simulink model "xblock_half_band_Model"  (Simulink 7.4)
settings: Solver=ode45  StartTime=0.0  StopTime=10.0  RelTol=1e-3
libraries: xbsIndex_r4 x629, casper_library_misc x12
(part 2 of 6)

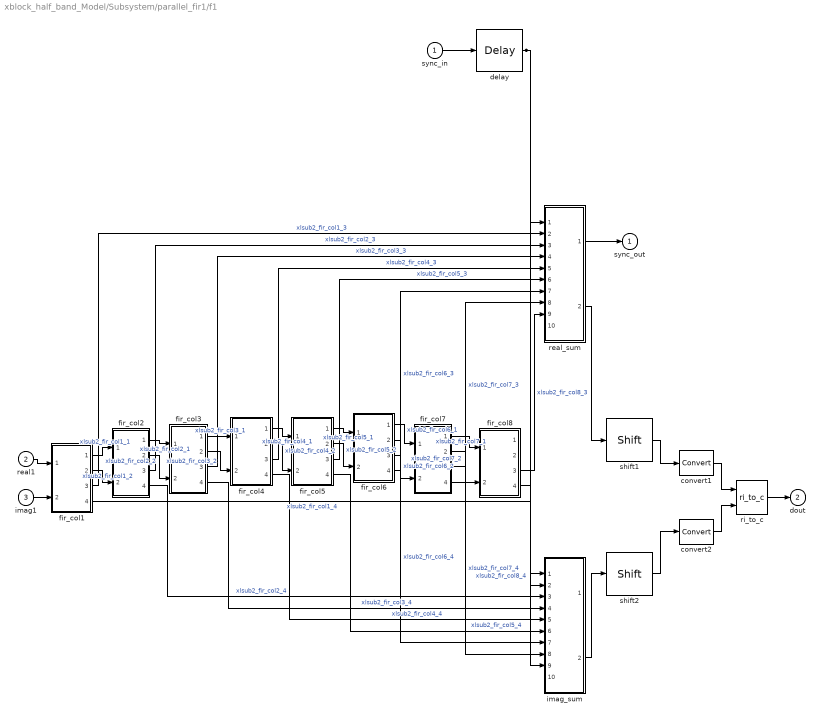
== system xblock_half_band_Model/Subsystem/parallel_fir1/f1 ==
  sync_in : Inport
  real1 : Inport  Port=2
  imag1 : Inport  Port=3
  convert1 : xbsIndex_r4/Convert  arith_type="Signed  (2's comp)"  n_bits=4  bin_pt=3  quantization=Truncate  overflow=Wrap  latency=1  dbl_ovrd=off  pipeline=off  block_type=convert
      settings: block_version=11.4
  convert2 : xbsIndex_r4/Convert  arith_type="Signed  (2's comp)"  n_bits=4  bin_pt=3  quantization=Truncate  overflow=Wrap  latency=1  dbl_ovrd=off  pipeline=off  block_type=convert
      settings: block_version=11.4
  delay : xbsIndex_r4/Delay  en=off  latency=3  dbl_ovrd=off  reg_retiming=off  block_type=delay
      settings: block_version=11.4
  fir_col1 : Subsystem
  fir_col2 : Subsystem
  fir_col3 : Subsystem
  fir_col4 : Subsystem
  fir_col5 : Subsystem
  fir_col6 : Subsystem
  fir_col7 : Subsystem
  fir_col8 : Subsystem
  imag_sum : Subsystem
  real_sum : Subsystem
  ri_to_c : casper_library_misc/ri_to_c  SystemSampleTime=-1
  shift1 : xbsIndex_r4/Shift  shift_dir=Left  shift_bits=1  en=off  latency=0  precision=Full  arith_type="Signed  (2's comp)"  n_bits=16  bin_pt=14  quantization=Truncate  overflow=Wrap  dbl_ovrd=off  block_type=shift
  shift2 : xbsIndex_r4/Shift  shift_dir=Left  shift_bits=1  en=off  latency=0  precision=Full  arith_type="Signed  (2's comp)"  n_bits=16  bin_pt=14  quantization=Truncate  overflow=Wrap  dbl_ovrd=off  block_type=shift
  sync_out : Outport
  dout : Outport  Port=2
  wires:
  delay/1 -> real_sum/1(sync), imag_sum/1(sync)
  imag_sum/2(dout) -> shift2/1
  shift1/1 -> convert1/1
  convert2/1 -> ri_to_c/2
  fir_col8/3(real_sum) -> real_sum/9(din_8)  "xlsub2_fir_col8_3"
  fir_col6/3(real_sum) -> real_sum/7(din_6)  "xlsub2_fir_col6_3"
  fir_col4/3(real_sum) -> real_sum/5(din_4)  "xlsub2_fir_col4_3"
  fir_col2/3(real_sum) -> real_sum/3(din_2)  "xlsub2_fir_col2_3"
  fir_col8/4(imag_sum) -> imag_sum/9(din_8)  "xlsub2_fir_col8_4"
  fir_col6/4(imag_sum) -> imag_sum/7(din_6)  "xlsub2_fir_col6_4"
  fir_col4/4(imag_sum) -> imag_sum/5(din_4)  "xlsub2_fir_col4_4"
  fir_col2/4(imag_sum) -> imag_sum/3(din_2)  "xlsub2_fir_col2_4"
  fir_col7/2(imag_out1) -> fir_col8/2(imag1)  "xlsub2_fir_col7_2"
  fir_col6/1(real_out1) -> fir_col7/1(real1)  "xlsub2_fir_col6_1"
  fir_col5/2(imag_out1) -> fir_col6/2(imag1)  "xlsub2_fir_col5_2"
  fir_col4/1(real_out1) -> fir_col5/1(real1)  "xlsub2_fir_col4_1"
  fir_col3/2(imag_out1) -> fir_col4/2(imag1)  "xlsub2_fir_col3_2"
  fir_col2/1(real_out1) -> fir_col3/1(real1)  "xlsub2_fir_col2_1"
  fir_col1/2(imag_out1) -> fir_col2/2(imag1)  "xlsub2_fir_col1_2"
  real1/1 -> fir_col1/1(real1)
  sync_in/1 -> delay/1
  imag1/1 -> fir_col1/2(imag1)
  fir_col1/1(real_out1) -> fir_col2/1(real1)  "xlsub2_fir_col1_1"
  fir_col2/2(imag_out1) -> fir_col3/2(imag1)  "xlsub2_fir_col2_2"
  fir_col3/1(real_out1) -> fir_col4/1(real1)  "xlsub2_fir_col3_1"
  fir_col4/2(imag_out1) -> fir_col5/2(imag1)  "xlsub2_fir_col4_2"
  fir_col5/1(real_out1) -> fir_col6/1(real1)  "xlsub2_fir_col5_1"
  fir_col6/2(imag_out1) -> fir_col7/2(imag1)  "xlsub2_fir_col6_2"
  fir_col7/1(real_out1) -> fir_col8/1(real1)  "xlsub2_fir_col7_1"
  fir_col1/4(imag_sum) -> imag_sum/2(din_1)  "xlsub2_fir_col1_4"
  fir_col3/4(imag_sum) -> imag_sum/4(din_3)  "xlsub2_fir_col3_4"
  fir_col5/4(imag_sum) -> imag_sum/6(din_5)  "xlsub2_fir_col5_4"
  fir_col7/4(imag_sum) -> imag_sum/8(din_7)  "xlsub2_fir_col7_4"
  fir_col1/3(real_sum) -> real_sum/2(din_1)  "xlsub2_fir_col1_3"
  fir_col3/3(real_sum) -> real_sum/4(din_3)  "xlsub2_fir_col3_3"
  fir_col5/3(real_sum) -> real_sum/6(din_5)  "xlsub2_fir_col5_3"
  fir_col7/3(real_sum) -> real_sum/8(din_7)  "xlsub2_fir_col7_3"
  real_sum/1(sync_out) -> sync_out/1
  convert1/1 -> ri_to_c/1
  ri_to_c/1 -> dout/1
  real_sum/2(dout) -> shift1/1
  shift2/1 -> convert2/1

== system xblock_half_band_Model/Subsystem/parallel_fir2/c_to_ri ==
  c : Inport
  force_im : xbsIndex_r4/Reinterpret  force_arith_type=on  arith_type="Signed  (2's comp)"  force_bin_pt=on  bin_pt=7  block_type=reinterpret
      settings: infoedit="Changes signal type without altering the binary representation.   You can changed the signal between signed and unsigned, and relocate the binary point.<br><br>Hardware notes: In hardware this block costs nothing.<br><br>Example:  Suppose the input is 6 bits wide, signed, with 2 fractional bits, and the output is forced to unsigned with 0 fractional bits.  Then an input of -2.0 (1110.00 in binary 2's complement) becomes an output of 56 (111000 in binary)."
  force_re : xbsIndex_r4/Reinterpret  force_arith_type=on  arith_type="Signed  (2's comp)"  force_bin_pt=on  bin_pt=7  block_type=reinterpret
      settings: infoedit="Changes signal type without altering the binary representation.   You can changed the signal between signed and unsigned, and relocate the binary point.<br><br>Hardware notes: In hardware this block costs nothing.<br><br>Example:  Suppose the input is 6 bits wide, signed, with 2 fractional bits, and the output is forced to unsigned with 0 fractional bits.  Then an input of -2.0 (1110.00 in binary 2's complement) becomes an output of 56 (111000 in binary)."
  slice_im : xbsIndex_r4/Slice  nbits=8  boolean_output=off  mode=Lower Bit Location + Width  bit1=0  base1=MSB of Input  bit0=0  base0=LSB of Input  dbl_ovrd=off  block_type=slice
  slice_re : xbsIndex_r4/Slice  nbits=8  boolean_output=off  mode=Upper Bit Location + Width  bit1=0  base1=MSB of Input  bit0=0  base0=LSB of Input  dbl_ovrd=off  block_type=slice
  re : Outport
  im : Outport  Port=2
  wires:
  c/1 -> slice_re/1, slice_im/1
  slice_im/1 -> force_im/1
  force_im/1 -> im/1
  force_re/1 -> re/1
  slice_re/1 -> force_re/1

== system xblock_half_band_Model/Subsystem/parallel_fir2/c_to_ri1 ==
  c : Inport
  force_im : xbsIndex_r4/Reinterpret  force_arith_type=on  arith_type="Signed  (2's comp)"  force_bin_pt=on  bin_pt=7  block_type=reinterpret
      settings: infoedit="Changes signal type without altering the binary representation.   You can changed the signal between signed and unsigned, and relocate the binary point.<br><br>Hardware notes: In hardware this block costs nothing.<br><br>Example:  Suppose the input is 6 bits wide, signed, with 2 fractional bits, and the output is forced to unsigned with 0 fractional bits.  Then an input of -2.0 (1110.00 in binary 2's complement) becomes an output of 56 (111000 in binary)."
  force_re : xbsIndex_r4/Reinterpret  force_arith_type=on  arith_type="Signed  (2's comp)"  force_bin_pt=on  bin_pt=7  block_type=reinterpret
      settings: infoedit="Changes signal type without altering the binary representation.   You can changed the signal between signed and unsigned, and relocate the binary point.<br><br>Hardware notes: In hardware this block costs nothing.<br><br>Example:  Suppose the input is 6 bits wide, signed, with 2 fractional bits, and the output is forced to unsigned with 0 fractional bits.  Then an input of -2.0 (1110.00 in binary 2's complement) becomes an output of 56 (111000 in binary)."
  slice_im : xbsIndex_r4/Slice  nbits=8  boolean_output=off  mode=Lower Bit Location + Width  bit1=0  base1=MSB of Input  bit0=0  base0=LSB of Input  dbl_ovrd=off  block_type=slice
  slice_re : xbsIndex_r4/Slice  nbits=8  boolean_output=off  mode=Upper Bit Location + Width  bit1=0  base1=MSB of Input  bit0=0  base0=LSB of Input  dbl_ovrd=off  block_type=slice
  re : Outport
  im : Outport  Port=2
  wires:
  c/1 -> slice_re/1, slice_im/1
  slice_im/1 -> force_im/1
  force_im/1 -> im/1
  force_re/1 -> re/1
  slice_re/1 -> force_re/1

== system xblock_half_band_Model/Subsystem/parallel_fir2/c_to_ri2 ==
  c : Inport
  force_im : xbsIndex_r4/Reinterpret  force_arith_type=on  arith_type="Signed  (2's comp)"  force_bin_pt=on  bin_pt=7  block_type=reinterpret
      settings: infoedit="Changes signal type without altering the binary representation.   You can changed the signal between signed and unsigned, and relocate the binary point.<br><br>Hardware notes: In hardware this block costs nothing.<br><br>Example:  Suppose the input is 6 bits wide, signed, with 2 fractional bits, and the output is forced to unsigned with 0 fractional bits.  Then an input of -2.0 (1110.00 in binary 2's complement) becomes an output of 56 (111000 in binary)."
  force_re : xbsIndex_r4/Reinterpret  force_arith_type=on  arith_type="Signed  (2's comp)"  force_bin_pt=on  bin_pt=7  block_type=reinterpret
      settings: infoedit="Changes signal type without altering the binary representation.   You can changed the signal between signed and unsigned, and relocate the binary point.<br><br>Hardware notes: In hardware this block costs nothing.<br><br>Example:  Suppose the input is 6 bits wide, signed, with 2 fractional bits, and the output is forced to unsigned with 0 fractional bits.  Then an input of -2.0 (1110.00 in binary 2's complement) becomes an output of 56 (111000 in binary)."
  slice_im : xbsIndex_r4/Slice  nbits=8  boolean_output=off  mode=Lower Bit Location + Width  bit1=0  base1=MSB of Input  bit0=0  base0=LSB of Input  dbl_ovrd=off  block_type=slice
  slice_re : xbsIndex_r4/Slice  nbits=8  boolean_output=off  mode=Upper Bit Location + Width  bit1=0  base1=MSB of Input  bit0=0  base0=LSB of Input  dbl_ovrd=off  block_type=slice
  re : Outport
  im : Outport  Port=2
  wires:
  c/1 -> slice_re/1, slice_im/1
  slice_im/1 -> force_im/1
  force_im/1 -> im/1
  force_re/1 -> re/1
  slice_re/1 -> force_re/1

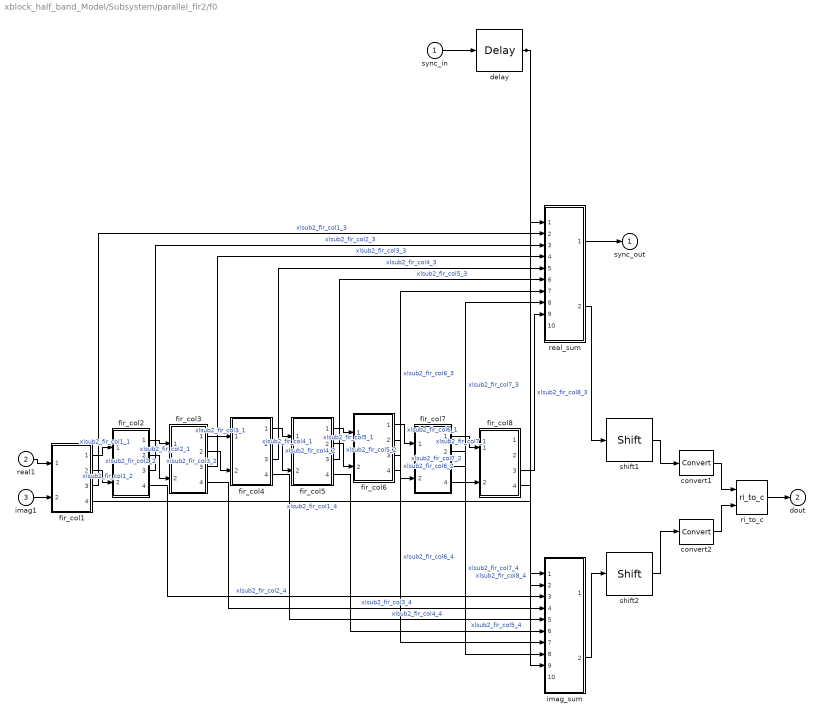
== system xblock_half_band_Model/Subsystem/parallel_fir2/f0 ==
  sync_in : Inport
  real1 : Inport  Port=2
  imag1 : Inport  Port=3
  convert1 : xbsIndex_r4/Convert  arith_type="Signed  (2's comp)"  n_bits=4  bin_pt=3  quantization=Truncate  overflow=Wrap  latency=1  dbl_ovrd=off  pipeline=off  block_type=convert
      settings: block_version=11.4
  convert2 : xbsIndex_r4/Convert  arith_type="Signed  (2's comp)"  n_bits=4  bin_pt=3  quantization=Truncate  overflow=Wrap  latency=1  dbl_ovrd=off  pipeline=off  block_type=convert
      settings: block_version=11.4
  delay : xbsIndex_r4/Delay  en=off  latency=3  dbl_ovrd=off  reg_retiming=off  block_type=delay
      settings: block_version=11.4
  fir_col1 : Subsystem
  fir_col2 : Subsystem
  fir_col3 : Subsystem
  fir_col4 : Subsystem
  fir_col5 : Subsystem
  fir_col6 : Subsystem
  fir_col7 : Subsystem
  fir_col8 : Subsystem
  imag_sum : Subsystem
  real_sum : Subsystem
  ri_to_c : casper_library_misc/ri_to_c  SystemSampleTime=-1
  shift1 : xbsIndex_r4/Shift  shift_dir=Left  shift_bits=1  en=off  latency=0  precision=Full  arith_type="Signed  (2's comp)"  n_bits=16  bin_pt=14  quantization=Truncate  overflow=Wrap  dbl_ovrd=off  block_type=shift
  shift2 : xbsIndex_r4/Shift  shift_dir=Left  shift_bits=1  en=off  latency=0  precision=Full  arith_type="Signed  (2's comp)"  n_bits=16  bin_pt=14  quantization=Truncate  overflow=Wrap  dbl_ovrd=off  block_type=shift
  sync_out : Outport
  dout : Outport  Port=2
  wires:
  delay/1 -> real_sum/1(sync), imag_sum/1(sync)
  imag_sum/2(dout) -> shift2/1
  shift1/1 -> convert1/1
  convert2/1 -> ri_to_c/2
  fir_col8/3(real_sum) -> real_sum/9(din_8)  "xlsub2_fir_col8_3"
  fir_col6/3(real_sum) -> real_sum/7(din_6)  "xlsub2_fir_col6_3"
  fir_col4/3(real_sum) -> real_sum/5(din_4)  "xlsub2_fir_col4_3"
  fir_col2/3(real_sum) -> real_sum/3(din_2)  "xlsub2_fir_col2_3"
  fir_col8/4(imag_sum) -> imag_sum/9(din_8)  "xlsub2_fir_col8_4"
  fir_col6/4(imag_sum) -> imag_sum/7(din_6)  "xlsub2_fir_col6_4"
  fir_col4/4(imag_sum) -> imag_sum/5(din_4)  "xlsub2_fir_col4_4"
  fir_col2/4(imag_sum) -> imag_sum/3(din_2)  "xlsub2_fir_col2_4"
  fir_col7/2(imag_out1) -> fir_col8/2(imag1)  "xlsub2_fir_col7_2"
  fir_col6/1(real_out1) -> fir_col7/1(real1)  "xlsub2_fir_col6_1"
  fir_col5/2(imag_out1) -> fir_col6/2(imag1)  "xlsub2_fir_col5_2"
  fir_col4/1(real_out1) -> fir_col5/1(real1)  "xlsub2_fir_col4_1"
  fir_col3/2(imag_out1) -> fir_col4/2(imag1)  "xlsub2_fir_col3_2"
  fir_col2/1(real_out1) -> fir_col3/1(real1)  "xlsub2_fir_col2_1"
  fir_col1/2(imag_out1) -> fir_col2/2(imag1)  "xlsub2_fir_col1_2"
  real1/1 -> fir_col1/1(real1)
  sync_in/1 -> delay/1
  imag1/1 -> fir_col1/2(imag1)
  fir_col1/1(real_out1) -> fir_col2/1(real1)  "xlsub2_fir_col1_1"
  fir_col2/2(imag_out1) -> fir_col3/2(imag1)  "xlsub2_fir_col2_2"
  fir_col3/1(real_out1) -> fir_col4/1(real1)  "xlsub2_fir_col3_1"
  fir_col4/2(imag_out1) -> fir_col5/2(imag1)  "xlsub2_fir_col4_2"
  fir_col5/1(real_out1) -> fir_col6/1(real1)  "xlsub2_fir_col5_1"
  fir_col6/2(imag_out1) -> fir_col7/2(imag1)  "xlsub2_fir_col6_2"
  fir_col7/1(real_out1) -> fir_col8/1(real1)  "xlsub2_fir_col7_1"
  fir_col1/4(imag_sum) -> imag_sum/2(din_1)  "xlsub2_fir_col1_4"
  fir_col3/4(imag_sum) -> imag_sum/4(din_3)  "xlsub2_fir_col3_4"
  fir_col5/4(imag_sum) -> imag_sum/6(din_5)  "xlsub2_fir_col5_4"
  fir_col7/4(imag_sum) -> imag_sum/8(din_7)  "xlsub2_fir_col7_4"
  fir_col1/3(real_sum) -> real_sum/2(din_1)  "xlsub2_fir_col1_3"
  fir_col3/3(real_sum) -> real_sum/4(din_3)  "xlsub2_fir_col3_3"
  fir_col5/3(real_sum) -> real_sum/6(din_5)  "xlsub2_fir_col5_3"
  fir_col7/3(real_sum) -> real_sum/8(din_7)  "xlsub2_fir_col7_3"
  real_sum/1(sync_out) -> sync_out/1
  convert1/1 -> ri_to_c/1
  ri_to_c/1 -> dout/1
  real_sum/2(dout) -> shift1/1
  shift2/1 -> convert2/1

== system xblock_half_band_Model/Subsystem/parallel_fir2/f0pf1 ==
  sync_in : Inport
  real1 : Inport  Port=2
  imag1 : Inport  Port=3
  convert1 : xbsIndex_r4/Convert  arith_type="Signed  (2's comp)"  n_bits=4  bin_pt=3  quantization=Truncate  overflow=Wrap  latency=1  dbl_ovrd=off  pipeline=off  block_type=convert
      settings: block_version=11.4
  convert2 : xbsIndex_r4/Convert  arith_type="Signed  (2's comp)"  n_bits=4  bin_pt=3  quantization=Truncate  overflow=Wrap  latency=1  dbl_ovrd=off  pipeline=off  block_type=convert
      settings: block_version=11.4
  delay : xbsIndex_r4/Delay  en=off  latency=3  dbl_ovrd=off  reg_retiming=off  block_type=delay
      settings: block_version=11.4
  fir_col1 : Subsystem
  fir_col2 : Subsystem
  fir_col3 : Subsystem
  fir_col4 : Subsystem
  fir_col5 : Subsystem
  imag_sum : Subsystem
  real_sum : Subsystem
  ri_to_c : casper_library_misc/ri_to_c  SystemSampleTime=-1
  shift1 : xbsIndex_r4/Shift  shift_dir=Left  shift_bits=1  en=off  latency=0  precision=Full  arith_type="Signed  (2's comp)"  n_bits=16  bin_pt=14  quantization=Truncate  overflow=Wrap  dbl_ovrd=off  block_type=shift
  shift2 : xbsIndex_r4/Shift  shift_dir=Left  shift_bits=1  en=off  latency=0  precision=Full  arith_type="Signed  (2's comp)"  n_bits=16  bin_pt=14  quantization=Truncate  overflow=Wrap  dbl_ovrd=off  block_type=shift
  sync_out : Outport
  dout : Outport  Port=2
  wires:
  delay/1 -> imag_sum/1(sync), real_sum/1(sync)
  imag_sum/2(dout) -> shift2/1
  shift1/1 -> convert1/1
  convert2/1 -> ri_to_c/2
  fir_col5/3(real_sum) -> real_sum/6(din_5)  "xlsub2_fir_col5_3"
  fir_col3/3(real_sum) -> real_sum/4(din_3)  "xlsub2_fir_col3_3"
  fir_col1/3(real_sum) -> real_sum/2(din_1)  "xlsub2_fir_col1_3"
  fir_col4/4(imag_sum) -> imag_sum/5(din_4)  "xlsub2_fir_col4_4"
  fir_col2/4(imag_sum) -> imag_sum/3(din_2)  "xlsub2_fir_col2_4"
  fir_col4/2(imag_out1) -> fir_col5/2(imag1)  "xlsub2_fir_col4_2"
  fir_col3/1(real_out1) -> fir_col4/1(real1)  "xlsub2_fir_col3_1"
  fir_col2/2(imag_out1) -> fir_col3/2(imag1)  "xlsub2_fir_col2_2"
  fir_col1/1(real_out1) -> fir_col2/1(real1)  "xlsub2_fir_col1_1"
  imag1/1 -> fir_col1/2(imag1)
  sync_in/1 -> delay/1
  real1/1 -> fir_col1/1(real1)
  fir_col1/2(imag_out1) -> fir_col2/2(imag1)  "xlsub2_fir_col1_2"
  fir_col2/1(real_out1) -> fir_col3/1(real1)  "xlsub2_fir_col2_1"
  fir_col3/2(imag_out1) -> fir_col4/2(imag1)  "xlsub2_fir_col3_2"
  fir_col4/1(real_out1) -> fir_col5/1(real1)  "xlsub2_fir_col4_1"
  fir_col1/4(imag_sum) -> imag_sum/2(din_1)  "xlsub2_fir_col1_4"
  fir_col3/4(imag_sum) -> imag_sum/4(din_3)  "xlsub2_fir_col3_4"
  fir_col5/4(imag_sum) -> imag_sum/6(din_5)  "xlsub2_fir_col5_4"
  fir_col2/3(real_sum) -> real_sum/3(din_2)  "xlsub2_fir_col2_3"
  fir_col4/3(real_sum) -> real_sum/5(din_4)  "xlsub2_fir_col4_3"
  real_sum/1(sync_out) -> sync_out/1
  convert1/1 -> ri_to_c/1
  ri_to_c/1 -> dout/1
  real_sum/2(dout) -> shift1/1
  shift2/1 -> convert2/1

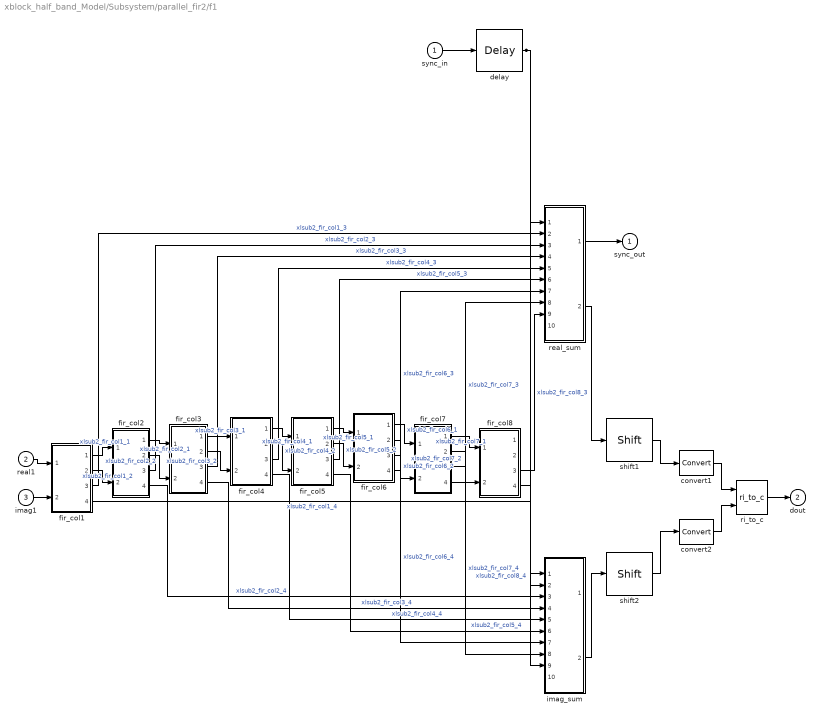
== system xblock_half_band_Model/Subsystem/parallel_fir2/f1 ==
  sync_in : Inport
  real1 : Inport  Port=2
  imag1 : Inport  Port=3
  convert1 : xbsIndex_r4/Convert  arith_type="Signed  (2's comp)"  n_bits=4  bin_pt=3  quantization=Truncate  overflow=Wrap  latency=1  dbl_ovrd=off  pipeline=off  block_type=convert
      settings: block_version=11.4
  convert2 : xbsIndex_r4/Convert  arith_type="Signed  (2's comp)"  n_bits=4  bin_pt=3  quantization=Truncate  overflow=Wrap  latency=1  dbl_ovrd=off  pipeline=off  block_type=convert
      settings: block_version=11.4
  delay : xbsIndex_r4/Delay  en=off  latency=3  dbl_ovrd=off  reg_retiming=off  block_type=delay
      settings: block_version=11.4
  fir_col1 : Subsystem
  fir_col2 : Subsystem
  fir_col3 : Subsystem
  fir_col4 : Subsystem
  fir_col5 : Subsystem
  fir_col6 : Subsystem
  fir_col7 : Subsystem
  fir_col8 : Subsystem
  imag_sum : Subsystem
  real_sum : Subsystem
  ri_to_c : casper_library_misc/ri_to_c  SystemSampleTime=-1
  shift1 : xbsIndex_r4/Shift  shift_dir=Left  shift_bits=1  en=off  latency=0  precision=Full  arith_type="Signed  (2's comp)"  n_bits=16  bin_pt=14  quantization=Truncate  overflow=Wrap  dbl_ovrd=off  block_type=shift
  shift2 : xbsIndex_r4/Shift  shift_dir=Left  shift_bits=1  en=off  latency=0  precision=Full  arith_type="Signed  (2's comp)"  n_bits=16  bin_pt=14  quantization=Truncate  overflow=Wrap  dbl_ovrd=off  block_type=shift
  sync_out : Outport
  dout : Outport  Port=2
  wires:
  delay/1 -> real_sum/1(sync), imag_sum/1(sync)
  imag_sum/2(dout) -> shift2/1
  shift1/1 -> convert1/1
  convert2/1 -> ri_to_c/2
  fir_col8/3(real_sum) -> real_sum/9(din_8)  "xlsub2_fir_col8_3"
  fir_col6/3(real_sum) -> real_sum/7(din_6)  "xlsub2_fir_col6_3"
  fir_col4/3(real_sum) -> real_sum/5(din_4)  "xlsub2_fir_col4_3"
  fir_col2/3(real_sum) -> real_sum/3(din_2)  "xlsub2_fir_col2_3"
  fir_col8/4(imag_sum) -> imag_sum/9(din_8)  "xlsub2_fir_col8_4"
  fir_col6/4(imag_sum) -> imag_sum/7(din_6)  "xlsub2_fir_col6_4"
  fir_col4/4(imag_sum) -> imag_sum/5(din_4)  "xlsub2_fir_col4_4"
  fir_col2/4(imag_sum) -> imag_sum/3(din_2)  "xlsub2_fir_col2_4"
  fir_col7/2(imag_out1) -> fir_col8/2(imag1)  "xlsub2_fir_col7_2"
  fir_col6/1(real_out1) -> fir_col7/1(real1)  "xlsub2_fir_col6_1"
  fir_col5/2(imag_out1) -> fir_col6/2(imag1)  "xlsub2_fir_col5_2"
  fir_col4/1(real_out1) -> fir_col5/1(real1)  "xlsub2_fir_col4_1"
  fir_col3/2(imag_out1) -> fir_col4/2(imag1)  "xlsub2_fir_col3_2"
  fir_col2/1(real_out1) -> fir_col3/1(real1)  "xlsub2_fir_col2_1"
  fir_col1/2(imag_out1) -> fir_col2/2(imag1)  "xlsub2_fir_col1_2"
  real1/1 -> fir_col1/1(real1)
  sync_in/1 -> delay/1
  imag1/1 -> fir_col1/2(imag1)
  fir_col1/1(real_out1) -> fir_col2/1(real1)  "xlsub2_fir_col1_1"
  fir_col2/2(imag_out1) -> fir_col3/2(imag1)  "xlsub2_fir_col2_2"
  fir_col3/1(real_out1) -> fir_col4/1(real1)  "xlsub2_fir_col3_1"
  fir_col4/2(imag_out1) -> fir_col5/2(imag1)  "xlsub2_fir_col4_2"
  fir_col5/1(real_out1) -> fir_col6/1(real1)  "xlsub2_fir_col5_1"
  fir_col6/2(imag_out1) -> fir_col7/2(imag1)  "xlsub2_fir_col6_2"
  fir_col7/1(real_out1) -> fir_col8/1(real1)  "xlsub2_fir_col7_1"
  fir_col1/4(imag_sum) -> imag_sum/2(din_1)  "xlsub2_fir_col1_4"
  fir_col3/4(imag_sum) -> imag_sum/4(din_3)  "xlsub2_fir_col3_4"
  fir_col5/4(imag_sum) -> imag_sum/6(din_5)  "xlsub2_fir_col5_4"
  fir_col7/4(imag_sum) -> imag_sum/8(din_7)  "xlsub2_fir_col7_4"
  fir_col1/3(real_sum) -> real_sum/2(din_1)  "xlsub2_fir_col1_3"
  fir_col3/3(real_sum) -> real_sum/4(din_3)  "xlsub2_fir_col3_3"
  fir_col5/3(real_sum) -> real_sum/6(din_5)  "xlsub2_fir_col5_3"
  fir_col7/3(real_sum) -> real_sum/8(din_7)  "xlsub2_fir_col7_3"
  real_sum/1(sync_out) -> sync_out/1
  convert1/1 -> ri_to_c/1
  ri_to_c/1 -> dout/1
  real_sum/2(dout) -> shift1/1
  shift2/1 -> convert2/1

== system xblock_half_band_Model/Subsystem/parallel_fir3/c_to_ri ==
  c : Inport
  force_im : xbsIndex_r4/Reinterpret  force_arith_type=on  arith_type="Signed  (2's comp)"  force_bin_pt=on  bin_pt=7  block_type=reinterpret
      settings: infoedit="Changes signal type without altering the binary representation.   You can changed the signal between signed and unsigned, and relocate the binary point.<br><br>Hardware notes: In hardware this block costs nothing.<br><br>Example:  Suppose the input is 6 bits wide, signed, with 2 fractional bits, and the output is forced to unsigned with 0 fractional bits.  Then an input of -2.0 (1110.00 in binary 2's complement) becomes an output of 56 (111000 in binary)."
  force_re : xbsIndex_r4/Reinterpret  force_arith_type=on  arith_type="Signed  (2's comp)"  force_bin_pt=on  bin_pt=7  block_type=reinterpret
      settings: infoedit="Changes signal type without altering the binary representation.   You can changed the signal between signed and unsigned, and relocate the binary point.<br><br>Hardware notes: In hardware this block costs nothing.<br><br>Example:  Suppose the input is 6 bits wide, signed, with 2 fractional bits, and the output is forced to unsigned with 0 fractional bits.  Then an input of -2.0 (1110.00 in binary 2's complement) becomes an output of 56 (111000 in binary)."
  slice_im : xbsIndex_r4/Slice  nbits=8  boolean_output=off  mode=Lower Bit Location + Width  bit1=0  base1=MSB of Input  bit0=0  base0=LSB of Input  dbl_ovrd=off  block_type=slice
  slice_re : xbsIndex_r4/Slice  nbits=8  boolean_output=off  mode=Upper Bit Location + Width  bit1=0  base1=MSB of Input  bit0=0  base0=LSB of Input  dbl_ovrd=off  block_type=slice
  re : Outport
  im : Outport  Port=2
  wires:
  c/1 -> slice_re/1, slice_im/1
  slice_im/1 -> force_im/1
  force_im/1 -> im/1
  force_re/1 -> re/1
  slice_re/1 -> force_re/1

== system xblock_half_band_Model/Subsystem/parallel_fir3/c_to_ri1 ==
  c : Inport
  force_im : xbsIndex_r4/Reinterpret  force_arith_type=on  arith_type="Signed  (2's comp)"  force_bin_pt=on  bin_pt=7  block_type=reinterpret
      settings: infoedit="Changes signal type without altering the binary representation.   You can changed the signal between signed and unsigned, and relocate the binary point.<br><br>Hardware notes: In hardware this block costs nothing.<br><br>Example:  Suppose the input is 6 bits wide, signed, with 2 fractional bits, and the output is forced to unsigned with 0 fractional bits.  Then an input of -2.0 (1110.00 in binary 2's complement) becomes an output of 56 (111000 in binary)."
  force_re : xbsIndex_r4/Reinterpret  force_arith_type=on  arith_type="Signed  (2's comp)"  force_bin_pt=on  bin_pt=7  block_type=reinterpret
      settings: infoedit="Changes signal type without altering the binary representation.   You can changed the signal between signed and unsigned, and relocate the binary point.<br><br>Hardware notes: In hardware this block costs nothing.<br><br>Example:  Suppose the input is 6 bits wide, signed, with 2 fractional bits, and the output is forced to unsigned with 0 fractional bits.  Then an input of -2.0 (1110.00 in binary 2's complement) becomes an output of 56 (111000 in binary)."
  slice_im : xbsIndex_r4/Slice  nbits=8  boolean_output=off  mode=Lower Bit Location + Width  bit1=0  base1=MSB of Input  bit0=0  base0=LSB of Input  dbl_ovrd=off  block_type=slice
  slice_re : xbsIndex_r4/Slice  nbits=8  boolean_output=off  mode=Upper Bit Location + Width  bit1=0  base1=MSB of Input  bit0=0  base0=LSB of Input  dbl_ovrd=off  block_type=slice
  re : Outport
  im : Outport  Port=2
  wires:
  c/1 -> slice_re/1, slice_im/1
  slice_im/1 -> force_im/1
  force_im/1 -> im/1
  force_re/1 -> re/1
  slice_re/1 -> force_re/1

== system xblock_half_band_Model/Subsystem/parallel_fir3/c_to_ri2 ==
  c : Inport
  force_im : xbsIndex_r4/Reinterpret  force_arith_type=on  arith_type="Signed  (2's comp)"  force_bin_pt=on  bin_pt=7  block_type=reinterpret
      settings: infoedit="Changes signal type without altering the binary representation.   You can changed the signal between signed and unsigned, and relocate the binary point.<br><br>Hardware notes: In hardware this block costs nothing.<br><br>Example:  Suppose the input is 6 bits wide, signed, with 2 fractional bits, and the output is forced to unsigned with 0 fractional bits.  Then an input of -2.0 (1110.00 in binary 2's complement) becomes an output of 56 (111000 in binary)."
  force_re : xbsIndex_r4/Reinterpret  force_arith_type=on  arith_type="Signed  (2's comp)"  force_bin_pt=on  bin_pt=7  block_type=reinterpret
      settings: infoedit="Changes signal type without altering the binary representation.   You can changed the signal between signed and unsigned, and relocate the binary point.<br><br>Hardware notes: In hardware this block costs nothing.<br><br>Example:  Suppose the input is 6 bits wide, signed, with 2 fractional bits, and the output is forced to unsigned with 0 fractional bits.  Then an input of -2.0 (1110.00 in binary 2's complement) becomes an output of 56 (111000 in binary)."
  slice_im : xbsIndex_r4/Slice  nbits=8  boolean_output=off  mode=Lower Bit Location + Width  bit1=0  base1=MSB of Input  bit0=0  base0=LSB of Input  dbl_ovrd=off  block_type=slice
  slice_re : xbsIndex_r4/Slice  nbits=8  boolean_output=off  mode=Upper Bit Location + Width  bit1=0  base1=MSB of Input  bit0=0  base0=LSB of Input  dbl_ovrd=off  block_type=slice
  re : Outport
  im : Outport  Port=2
  wires:
  c/1 -> slice_re/1, slice_im/1
  slice_im/1 -> force_im/1
  force_im/1 -> im/1
  force_re/1 -> re/1
  slice_re/1 -> force_re/1

== system xblock_half_band_Model/Subsystem/parallel_fir3/f0 ==
  sync_in : Inport
  real1 : Inport  Port=2
  imag1 : Inport  Port=3
  convert1 : xbsIndex_r4/Convert  arith_type="Signed  (2's comp)"  n_bits=4  bin_pt=3  quantization=Truncate  overflow=Wrap  latency=1  dbl_ovrd=off  pipeline=off  block_type=convert
      settings: block_version=11.4
  convert2 : xbsIndex_r4/Convert  arith_type="Signed  (2's comp)"  n_bits=4  bin_pt=3  quantization=Truncate  overflow=Wrap  latency=1  dbl_ovrd=off  pipeline=off  block_type=convert
      settings: block_version=11.4
  delay : xbsIndex_r4/Delay  en=off  latency=3  dbl_ovrd=off  reg_retiming=off  block_type=delay
      settings: block_version=11.4
  fir_col1 : Subsystem
  fir_col2 : Subsystem
  fir_col3 : Subsystem
  fir_col4 : Subsystem
  fir_col5 : Subsystem
  fir_col6 : Subsystem
  fir_col7 : Subsystem
  fir_col8 : Subsystem
  imag_sum : Subsystem
  real_sum : Subsystem
  ri_to_c : casper_library_misc/ri_to_c  SystemSampleTime=-1
  shift1 : xbsIndex_r4/Shift  shift_dir=Left  shift_bits=1  en=off  latency=0  precision=Full  arith_type="Signed  (2's comp)"  n_bits=16  bin_pt=14  quantization=Truncate  overflow=Wrap  dbl_ovrd=off  block_type=shift
  shift2 : xbsIndex_r4/Shift  shift_dir=Left  shift_bits=1  en=off  latency=0  precision=Full  arith_type="Signed  (2's comp)"  n_bits=16  bin_pt=14  quantization=Truncate  overflow=Wrap  dbl_ovrd=off  block_type=shift
  sync_out : Outport
  dout : Outport  Port=2
  wires:
  delay/1 -> real_sum/1(sync), imag_sum/1(sync)
  imag_sum/2(dout) -> shift2/1
  shift1/1 -> convert1/1
  convert2/1 -> ri_to_c/2
  fir_col8/3(real_sum) -> real_sum/9(din_8)  "xlsub2_fir_col8_3"
  fir_col6/3(real_sum) -> real_sum/7(din_6)  "xlsub2_fir_col6_3"
  fir_col4/3(real_sum) -> real_sum/5(din_4)  "xlsub2_fir_col4_3"
  fir_col2/3(real_sum) -> real_sum/3(din_2)  "xlsub2_fir_col2_3"
  fir_col8/4(imag_sum) -> imag_sum/9(din_8)  "xlsub2_fir_col8_4"
  fir_col6/4(imag_sum) -> imag_sum/7(din_6)  "xlsub2_fir_col6_4"
  fir_col4/4(imag_sum) -> imag_sum/5(din_4)  "xlsub2_fir_col4_4"
  fir_col2/4(imag_sum) -> imag_sum/3(din_2)  "xlsub2_fir_col2_4"
  fir_col7/2(imag_out1) -> fir_col8/2(imag1)  "xlsub2_fir_col7_2"
  fir_col6/1(real_out1) -> fir_col7/1(real1)  "xlsub2_fir_col6_1"
  fir_col5/2(imag_out1) -> fir_col6/2(imag1)  "xlsub2_fir_col5_2"
  fir_col4/1(real_out1) -> fir_col5/1(real1)  "xlsub2_fir_col4_1"
  fir_col3/2(imag_out1) -> fir_col4/2(imag1)  "xlsub2_fir_col3_2"
  fir_col2/1(real_out1) -> fir_col3/1(real1)  "xlsub2_fir_col2_1"
  fir_col1/2(imag_out1) -> fir_col2/2(imag1)  "xlsub2_fir_col1_2"
  real1/1 -> fir_col1/1(real1)
  sync_in/1 -> delay/1
  imag1/1 -> fir_col1/2(imag1)
  fir_col1/1(real_out1) -> fir_col2/1(real1)  "xlsub2_fir_col1_1"
  fir_col2/2(imag_out1) -> fir_col3/2(imag1)  "xlsub2_fir_col2_2"
  fir_col3/1(real_out1) -> fir_col4/1(real1)  "xlsub2_fir_col3_1"
  fir_col4/2(imag_out1) -> fir_col5/2(imag1)  "xlsub2_fir_col4_2"
  fir_col5/1(real_out1) -> fir_col6/1(real1)  "xlsub2_fir_col5_1"
  fir_col6/2(imag_out1) -> fir_col7/2(imag1)  "xlsub2_fir_col6_2"
  fir_col7/1(real_out1) -> fir_col8/1(real1)  "xlsub2_fir_col7_1"
  fir_col1/4(imag_sum) -> imag_sum/2(din_1)  "xlsub2_fir_col1_4"
  fir_col3/4(imag_sum) -> imag_sum/4(din_3)  "xlsub2_fir_col3_4"
  fir_col5/4(imag_sum) -> imag_sum/6(din_5)  "xlsub2_fir_col5_4"
  fir_col7/4(imag_sum) -> imag_sum/8(din_7)  "xlsub2_fir_col7_4"
  fir_col1/3(real_sum) -> real_sum/2(din_1)  "xlsub2_fir_col1_3"
  fir_col3/3(real_sum) -> real_sum/4(din_3)  "xlsub2_fir_col3_3"
  fir_col5/3(real_sum) -> real_sum/6(din_5)  "xlsub2_fir_col5_3"
  fir_col7/3(real_sum) -> real_sum/8(din_7)  "xlsub2_fir_col7_3"
  real_sum/1(sync_out) -> sync_out/1
  convert1/1 -> ri_to_c/1
  ri_to_c/1 -> dout/1
  real_sum/2(dout) -> shift1/1
  shift2/1 -> convert2/1

== system xblock_half_band_Model/Subsystem/parallel_fir3/f0pf1 ==
  sync_in : Inport
  real1 : Inport  Port=2
  imag1 : Inport  Port=3
  convert1 : xbsIndex_r4/Convert  arith_type="Signed  (2's comp)"  n_bits=4  bin_pt=3  quantization=Truncate  overflow=Wrap  latency=1  dbl_ovrd=off  pipeline=off  block_type=convert
      settings: block_version=11.4
  convert2 : xbsIndex_r4/Convert  arith_type="Signed  (2's comp)"  n_bits=4  bin_pt=3  quantization=Truncate  overflow=Wrap  latency=1  dbl_ovrd=off  pipeline=off  block_type=convert
      settings: block_version=11.4
  delay : xbsIndex_r4/Delay  en=off  latency=3  dbl_ovrd=off  reg_retiming=off  block_type=delay
      settings: block_version=11.4
  fir_col1 : Subsystem
  fir_col2 : Subsystem
  fir_col3 : Subsystem
  fir_col4 : Subsystem
  fir_col5 : Subsystem
  imag_sum : Subsystem
  real_sum : Subsystem
  ri_to_c : casper_library_misc/ri_to_c  SystemSampleTime=-1
  shift1 : xbsIndex_r4/Shift  shift_dir=Left  shift_bits=1  en=off  latency=0  precision=Full  arith_type="Signed  (2's comp)"  n_bits=16  bin_pt=14  quantization=Truncate  overflow=Wrap  dbl_ovrd=off  block_type=shift
  shift2 : xbsIndex_r4/Shift  shift_dir=Left  shift_bits=1  en=off  latency=0  precision=Full  arith_type="Signed  (2's comp)"  n_bits=16  bin_pt=14  quantization=Truncate  overflow=Wrap  dbl_ovrd=off  block_type=shift
  sync_out : Outport
  dout : Outport  Port=2
  wires:
  delay/1 -> imag_sum/1(sync), real_sum/1(sync)
  imag_sum/2(dout) -> shift2/1
  shift1/1 -> convert1/1
  convert2/1 -> ri_to_c/2
  fir_col5/3(real_sum) -> real_sum/6(din_5)  "xlsub2_fir_col5_3"
  fir_col3/3(real_sum) -> real_sum/4(din_3)  "xlsub2_fir_col3_3"
  fir_col1/3(real_sum) -> real_sum/2(din_1)  "xlsub2_fir_col1_3"
  fir_col4/4(imag_sum) -> imag_sum/5(din_4)  "xlsub2_fir_col4_4"
  fir_col2/4(imag_sum) -> imag_sum/3(din_2)  "xlsub2_fir_col2_4"
  fir_col4/2(imag_out1) -> fir_col5/2(imag1)  "xlsub2_fir_col4_2"
  fir_col3/1(real_out1) -> fir_col4/1(real1)  "xlsub2_fir_col3_1"
  fir_col2/2(imag_out1) -> fir_col3/2(imag1)  "xlsub2_fir_col2_2"
  fir_col1/1(real_out1) -> fir_col2/1(real1)  "xlsub2_fir_col1_1"
  imag1/1 -> fir_col1/2(imag1)
  sync_in/1 -> delay/1
  real1/1 -> fir_col1/1(real1)
  fir_col1/2(imag_out1) -> fir_col2/2(imag1)  "xlsub2_fir_col1_2"
  fir_col2/1(real_out1) -> fir_col3/1(real1)  "xlsub2_fir_col2_1"
  fir_col3/2(imag_out1) -> fir_col4/2(imag1)  "xlsub2_fir_col3_2"
  fir_col4/1(real_out1) -> fir_col5/1(real1)  "xlsub2_fir_col4_1"
  fir_col1/4(imag_sum) -> imag_sum/2(din_1)  "xlsub2_fir_col1_4"
  fir_col3/4(imag_sum) -> imag_sum/4(din_3)  "xlsub2_fir_col3_4"
  fir_col5/4(imag_sum) -> imag_sum/6(din_5)  "xlsub2_fir_col5_4"
  fir_col2/3(real_sum) -> real_sum/3(din_2)  "xlsub2_fir_col2_3"
  fir_col4/3(real_sum) -> real_sum/5(din_4)  "xlsub2_fir_col4_3"
  real_sum/1(sync_out) -> sync_out/1
  convert1/1 -> ri_to_c/1
  ri_to_c/1 -> dout/1
  real_sum/2(dout) -> shift1/1
  shift2/1 -> convert2/1

== system xblock_half_band_Model/Subsystem/parallel_fir3/f1 ==
  sync_in : Inport
  real1 : Inport  Port=2
  imag1 : Inport  Port=3
  convert1 : xbsIndex_r4/Convert  arith_type="Signed  (2's comp)"  n_bits=4  bin_pt=3  quantization=Truncate  overflow=Wrap  latency=1  dbl_ovrd=off  pipeline=off  block_type=convert
      settings: block_version=11.4
  convert2 : xbsIndex_r4/Convert  arith_type="Signed  (2's comp)"  n_bits=4  bin_pt=3  quantization=Truncate  overflow=Wrap  latency=1  dbl_ovrd=off  pipeline=off  block_type=convert
      settings: block_version=11.4
  delay : xbsIndex_r4/Delay  en=off  latency=3  dbl_ovrd=off  reg_retiming=off  block_type=delay
      settings: block_version=11.4
  fir_col1 : Subsystem
  fir_col2 : Subsystem
  fir_col3 : Subsystem
  fir_col4 : Subsystem
  fir_col5 : Subsystem
  fir_col6 : Subsystem
  fir_col7 : Subsystem
  fir_col8 : Subsystem
  imag_sum : Subsystem
  real_sum : Subsystem
  ri_to_c : casper_library_misc/ri_to_c  SystemSampleTime=-1
  shift1 : xbsIndex_r4/Shift  shift_dir=Left  shift_bits=1  en=off  latency=0  precision=Full  arith_type="Signed  (2's comp)"  n_bits=16  bin_pt=14  quantization=Truncate  overflow=Wrap  dbl_ovrd=off  block_type=shift
  shift2 : xbsIndex_r4/Shift  shift_dir=Left  shift_bits=1  en=off  latency=0  precision=Full  arith_type="Signed  (2's comp)"  n_bits=16  bin_pt=14  quantization=Truncate  overflow=Wrap  dbl_ovrd=off  block_type=shift
  sync_out : Outport
  dout : Outport  Port=2
  wires:
  delay/1 -> real_sum/1(sync), imag_sum/1(sync)
  imag_sum/2(dout) -> shift2/1
  shift1/1 -> convert1/1
  convert2/1 -> ri_to_c/2
  fir_col8/3(real_sum) -> real_sum/9(din_8)  "xlsub2_fir_col8_3"
  fir_col6/3(real_sum) -> real_sum/7(din_6)  "xlsub2_fir_col6_3"
  fir_col4/3(real_sum) -> real_sum/5(din_4)  "xlsub2_fir_col4_3"
  fir_col2/3(real_sum) -> real_sum/3(din_2)  "xlsub2_fir_col2_3"
  fir_col8/4(imag_sum) -> imag_sum/9(din_8)  "xlsub2_fir_col8_4"
  fir_col6/4(imag_sum) -> imag_sum/7(din_6)  "xlsub2_fir_col6_4"
  fir_col4/4(imag_sum) -> imag_sum/5(din_4)  "xlsub2_fir_col4_4"
  fir_col2/4(imag_sum) -> imag_sum/3(din_2)  "xlsub2_fir_col2_4"
  fir_col7/2(imag_out1) -> fir_col8/2(imag1)  "xlsub2_fir_col7_2"
  fir_col6/1(real_out1) -> fir_col7/1(real1)  "xlsub2_fir_col6_1"
  fir_col5/2(imag_out1) -> fir_col6/2(imag1)  "xlsub2_fir_col5_2"
  fir_col4/1(real_out1) -> fir_col5/1(real1)  "xlsub2_fir_col4_1"
  fir_col3/2(imag_out1) -> fir_col4/2(imag1)  "xlsub2_fir_col3_2"
  fir_col2/1(real_out1) -> fir_col3/1(real1)  "xlsub2_fir_col2_1"
  fir_col1/2(imag_out1) -> fir_col2/2(imag1)  "xlsub2_fir_col1_2"
  real1/1 -> fir_col1/1(real1)
  sync_in/1 -> delay/1
  imag1/1 -> fir_col1/2(imag1)
  fir_col1/1(real_out1) -> fir_col2/1(real1)  "xlsub2_fir_col1_1"
  fir_col2/2(imag_out1) -> fir_col3/2(imag1)  "xlsub2_fir_col2_2"
  fir_col3/1(real_out1) -> fir_col4/1(real1)  "xlsub2_fir_col3_1"
  fir_col4/2(imag_out1) -> fir_col5/2(imag1)  "xlsub2_fir_col4_2"
  fir_col5/1(real_out1) -> fir_col6/1(real1)  "xlsub2_fir_col5_1"
  fir_col6/2(imag_out1) -> fir_col7/2(imag1)  "xlsub2_fir_col6_2"
  fir_col7/1(real_out1) -> fir_col8/1(real1)  "xlsub2_fir_col7_1"
  fir_col1/4(imag_sum) -> imag_sum/2(din_1)  "xlsub2_fir_col1_4"
  fir_col3/4(imag_sum) -> imag_sum/4(din_3)  "xlsub2_fir_col3_4"
  fir_col5/4(imag_sum) -> imag_sum/6(din_5)  "xlsub2_fir_col5_4"
  fir_col7/4(imag_sum) -> imag_sum/8(din_7)  "xlsub2_fir_col7_4"
  fir_col1/3(real_sum) -> real_sum/2(din_1)  "xlsub2_fir_col1_3"
  fir_col3/3(real_sum) -> real_sum/4(din_3)  "xlsub2_fir_col3_3"
  fir_col5/3(real_sum) -> real_sum/6(din_5)  "xlsub2_fir_col5_3"
  fir_col7/3(real_sum) -> real_sum/8(din_7)  "xlsub2_fir_col7_3"
  real_sum/1(sync_out) -> sync_out/1
  convert1/1 -> ri_to_c/1
  ri_to_c/1 -> dout/1
  real_sum/2(dout) -> shift1/1
  shift2/1 -> convert2/1

== system xblock_half_band_Model/Subsystem/parallel_fir/f0/fir_col1 ==
  real1 : Inport
  imag1 : Inport  Port=2
  fir_tap1 : Subsystem
  real_out1 : Outport
  imag_out1 : Outport  Port=2
  real_sum : Outport  Port=3
  imag_sum : Outport  Port=4
  wires:
  fir_tap1/4(imag) -> imag_sum/1  "xlsub5_fir_tap1_image"
  fir_tap1/1(a_out) -> real_out1/1
  real1/1 -> fir_tap1/1(a)
  imag1/1 -> fir_tap1/2(b)
  fir_tap1/2(b_out) -> imag_out1/1
  fir_tap1/3(real) -> real_sum/1  "xlsub5_fir_tap1_real"

== system xblock_half_band_Model/Subsystem/parallel_fir/f0/fir_col2 ==
  real1 : Inport
  imag1 : Inport  Port=2
  fir_tap1 : Subsystem
  real_out1 : Outport
  imag_out1 : Outport  Port=2
  real_sum : Outport  Port=3
  imag_sum : Outport  Port=4
  wires:
  fir_tap1/4(imag) -> imag_sum/1  "xlsub5_fir_tap1_image"
  fir_tap1/1(a_out) -> real_out1/1
  real1/1 -> fir_tap1/1(a)
  imag1/1 -> fir_tap1/2(b)
  fir_tap1/2(b_out) -> imag_out1/1
  fir_tap1/3(real) -> real_sum/1  "xlsub5_fir_tap1_real"

== system xblock_half_band_Model/Subsystem/parallel_fir/f0/fir_col3 ==
  real1 : Inport
  imag1 : Inport  Port=2
  fir_tap1 : Subsystem
  real_out1 : Outport
  imag_out1 : Outport  Port=2
  real_sum : Outport  Port=3
  imag_sum : Outport  Port=4
  wires:
  fir_tap1/4(imag) -> imag_sum/1  "xlsub5_fir_tap1_image"
  fir_tap1/1(a_out) -> real_out1/1
  real1/1 -> fir_tap1/1(a)
  imag1/1 -> fir_tap1/2(b)
  fir_tap1/2(b_out) -> imag_out1/1
  fir_tap1/3(real) -> real_sum/1  "xlsub5_fir_tap1_real"

== system xblock_half_band_Model/Subsystem/parallel_fir/f0/fir_col4 ==
  real1 : Inport
  imag1 : Inport  Port=2
  fir_tap1 : Subsystem
  real_out1 : Outport
  imag_out1 : Outport  Port=2
  real_sum : Outport  Port=3
  imag_sum : Outport  Port=4
  wires:
  fir_tap1/4(imag) -> imag_sum/1  "xlsub5_fir_tap1_image"
  fir_tap1/1(a_out) -> real_out1/1
  real1/1 -> fir_tap1/1(a)
  imag1/1 -> fir_tap1/2(b)
  fir_tap1/2(b_out) -> imag_out1/1
  fir_tap1/3(real) -> real_sum/1  "xlsub5_fir_tap1_real"

== system xblock_half_band_Model/Subsystem/parallel_fir/f0/fir_col5 ==
  real1 : Inport
  imag1 : Inport  Port=2
  fir_tap1 : Subsystem
  real_out1 : Outport
  imag_out1 : Outport  Port=2
  real_sum : Outport  Port=3
  imag_sum : Outport  Port=4
  wires:
  fir_tap1/4(imag) -> imag_sum/1  "xlsub5_fir_tap1_image"
  fir_tap1/1(a_out) -> real_out1/1
  real1/1 -> fir_tap1/1(a)
  imag1/1 -> fir_tap1/2(b)
  fir_tap1/2(b_out) -> imag_out1/1
  fir_tap1/3(real) -> real_sum/1  "xlsub5_fir_tap1_real"

== system xblock_half_band_Model/Subsystem/parallel_fir/f0/fir_col6 ==
  real1 : Inport
  imag1 : Inport  Port=2
  fir_tap1 : Subsystem
  real_out1 : Outport
  imag_out1 : Outport  Port=2
  real_sum : Outport  Port=3
  imag_sum : Outport  Port=4
  wires:
  fir_tap1/4(imag) -> imag_sum/1  "xlsub5_fir_tap1_image"
  fir_tap1/1(a_out) -> real_out1/1
  real1/1 -> fir_tap1/1(a)
  imag1/1 -> fir_tap1/2(b)
  fir_tap1/2(b_out) -> imag_out1/1
  fir_tap1/3(real) -> real_sum/1  "xlsub5_fir_tap1_real"

== system xblock_half_band_Model/Subsystem/parallel_fir/f0/fir_col7 ==
  real1 : Inport
  imag1 : Inport  Port=2
  fir_tap1 : Subsystem
  real_out1 : Outport
  imag_out1 : Outport  Port=2
  real_sum : Outport  Port=3
  imag_sum : Outport  Port=4
  wires:
  fir_tap1/4(imag) -> imag_sum/1  "xlsub5_fir_tap1_image"
  fir_tap1/1(a_out) -> real_out1/1
  real1/1 -> fir_tap1/1(a)
  imag1/1 -> fir_tap1/2(b)
  fir_tap1/2(b_out) -> imag_out1/1
  fir_tap1/3(real) -> real_sum/1  "xlsub5_fir_tap1_real"

== system xblock_half_band_Model/Subsystem/parallel_fir/f0/fir_col8 ==
  real1 : Inport
  imag1 : Inport  Port=2
  fir_tap1 : Subsystem
  real_out1 : Outport
  imag_out1 : Outport  Port=2
  real_sum : Outport  Port=3
  imag_sum : Outport  Port=4
  wires:
  fir_tap1/4(imag) -> imag_sum/1  "xlsub5_fir_tap1_image"
  fir_tap1/1(a_out) -> real_out1/1
  real1/1 -> fir_tap1/1(a)
  imag1/1 -> fir_tap1/2(b)
  fir_tap1/2(b_out) -> imag_out1/1
  fir_tap1/3(real) -> real_sum/1  "xlsub5_fir_tap1_real"

== system xblock_half_band_Model/Subsystem/parallel_fir/f0/imag_sum ==
  sync : Inport
  din_1 : Inport  Port=2
  din_2 : Inport  Port=3
  din_3 : Inport  Port=4
  din_4 : Inport  Port=5
  din_5 : Inport  Port=6
  din_6 : Inport  Port=7
  din_7 : Inport  Port=8
  din_8 : Inport  Port=9
  din_9 : Inport  Port=10
  sync_delay : xbsIndex_r4/Delay  en=off  latency=4  dbl_ovrd=off  reg_retiming=off  block_type=delay
      settings: block_version=11.4
  zero_in : xbsIndex_r4/Constant  arith_type=Unsigned  const=0  n_bits=18  bin_pt=17  explicit_period=off  period=1  equ=P=C  opselect=C  inp2=PCIN>>17  opr=+  inp1=P  carry=CIN  dbl_ovrd=off  block_type=constant
      settings: block_version=11.4
  sync_out : Outport
  dout : Outport  Port=2
  wires:
  sync/1 -> sync_delay/1
  sync_delay/1 -> sync_out/1

== system xblock_half_band_Model/Subsystem/parallel_fir/f0/real_sum ==
  sync : Inport
  din_1 : Inport  Port=2
  din_2 : Inport  Port=3
  din_3 : Inport  Port=4
  din_4 : Inport  Port=5
  din_5 : Inport  Port=6
  din_6 : Inport  Port=7
  din_7 : Inport  Port=8
  din_8 : Inport  Port=9
  din_9 : Inport  Port=10
  sync_delay : xbsIndex_r4/Delay  en=off  latency=4  dbl_ovrd=off  reg_retiming=off  block_type=delay
      settings: block_version=11.4
  zero_in : xbsIndex_r4/Constant  arith_type=Unsigned  const=0  n_bits=18  bin_pt=17  explicit_period=off  period=1  equ=P=C  opselect=C  inp2=PCIN>>17  opr=+  inp1=P  carry=CIN  dbl_ovrd=off  block_type=constant
      settings: block_version=11.4
  sync_out : Outport
  dout : Outport  Port=2
  wires:
  sync/1 -> sync_delay/1
  sync_delay/1 -> sync_out/1

== system xblock_half_band_Model/Subsystem/parallel_fir/f0pf1/fir_col1 ==
  real1 : Inport
  imag1 : Inport  Port=2
  fir_tap1 : Subsystem
  real_out1 : Outport
  imag_out1 : Outport  Port=2
  real_sum : Outport  Port=3
  imag_sum : Outport  Port=4
  wires:
  fir_tap1/4(imag) -> imag_sum/1  "xlsub5_fir_tap1_image"
  fir_tap1/1(a_out) -> real_out1/1
  real1/1 -> fir_tap1/1(a)
  imag1/1 -> fir_tap1/2(b)
  fir_tap1/2(b_out) -> imag_out1/1
  fir_tap1/3(real) -> real_sum/1  "xlsub5_fir_tap1_real"

== system xblock_half_band_Model/Subsystem/parallel_fir/f0pf1/fir_col2 ==
  real1 : Inport
  imag1 : Inport  Port=2
  fir_tap1 : Subsystem
  real_out1 : Outport
  imag_out1 : Outport  Port=2
  real_sum : Outport  Port=3
  imag_sum : Outport  Port=4
  wires:
  fir_tap1/4(imag) -> imag_sum/1  "xlsub5_fir_tap1_image"
  fir_tap1/1(a_out) -> real_out1/1
  real1/1 -> fir_tap1/1(a)
  imag1/1 -> fir_tap1/2(b)
  fir_tap1/2(b_out) -> imag_out1/1
  fir_tap1/3(real) -> real_sum/1  "xlsub5_fir_tap1_real"

== system xblock_half_band_Model/Subsystem/parallel_fir/f0pf1/fir_col3 ==
  real1 : Inport
  imag1 : Inport  Port=2
  fir_tap1 : Subsystem
  real_out1 : Outport
  imag_out1 : Outport  Port=2
  real_sum : Outport  Port=3
  imag_sum : Outport  Port=4
  wires:
  fir_tap1/4(imag) -> imag_sum/1  "xlsub5_fir_tap1_image"
  fir_tap1/1(a_out) -> real_out1/1
  real1/1 -> fir_tap1/1(a)
  imag1/1 -> fir_tap1/2(b)
  fir_tap1/2(b_out) -> imag_out1/1
  fir_tap1/3(real) -> real_sum/1  "xlsub5_fir_tap1_real"

== system xblock_half_band_Model/Subsystem/parallel_fir/f0pf1/fir_col4 ==
  real1 : Inport
  imag1 : Inport  Port=2
  fir_tap1 : Subsystem
  real_out1 : Outport
  imag_out1 : Outport  Port=2
  real_sum : Outport  Port=3
  imag_sum : Outport  Port=4
  wires:
  fir_tap1/4(imag) -> imag_sum/1  "xlsub5_fir_tap1_image"
  fir_tap1/1(a_out) -> real_out1/1
  real1/1 -> fir_tap1/1(a)
  imag1/1 -> fir_tap1/2(b)
  fir_tap1/2(b_out) -> imag_out1/1
  fir_tap1/3(real) -> real_sum/1  "xlsub5_fir_tap1_real"

== system xblock_half_band_Model/Subsystem/parallel_fir/f0pf1/fir_col5 ==
  real1 : Inport
  imag1 : Inport  Port=2
  fir_tap1 : Subsystem
  real_out1 : Outport
  imag_out1 : Outport  Port=2
  real_sum : Outport  Port=3
  imag_sum : Outport  Port=4
  wires:
  fir_tap1/4(imag) -> imag_sum/1  "xlsub5_fir_tap1_image"
  fir_tap1/1(a_out) -> real_out1/1
  real1/1 -> fir_tap1/1(a)
  imag1/1 -> fir_tap1/2(b)
  fir_tap1/2(b_out) -> imag_out1/1
  fir_tap1/3(real) -> real_sum/1  "xlsub5_fir_tap1_real"

== system xblock_half_band_Model/Subsystem/parallel_fir/f0pf1/imag_sum ==
  sync : Inport
  din_1 : Inport  Port=2
  din_2 : Inport  Port=3
  din_3 : Inport  Port=4
  din_4 : Inport  Port=5
  din_5 : Inport  Port=6
  din_6 : Inport  Port=7
  sync_delay : xbsIndex_r4/Delay  en=off  latency=3  dbl_ovrd=off  reg_retiming=off  block_type=delay
      settings: block_version=11.4
  zero_in : xbsIndex_r4/Constant  arith_type=Unsigned  const=0  n_bits=18  bin_pt=17  explicit_period=off  period=1  equ=P=C  opselect=C  inp2=PCIN>>17  opr=+  inp1=P  carry=CIN  dbl_ovrd=off  block_type=constant
      settings: block_version=11.4
  sync_out : Outport
  dout : Outport  Port=2
  wires:
  sync/1 -> sync_delay/1
  sync_delay/1 -> sync_out/1

== system xblock_half_band_Model/Subsystem/parallel_fir/f0pf1/real_sum ==
  sync : Inport
  din_1 : Inport  Port=2
  din_2 : Inport  Port=3
  din_3 : Inport  Port=4
  din_4 : Inport  Port=5
  din_5 : Inport  Port=6
  din_6 : Inport  Port=7
  sync_delay : xbsIndex_r4/Delay  en=off  latency=3  dbl_ovrd=off  reg_retiming=off  block_type=delay
      settings: block_version=11.4
  zero_in : xbsIndex_r4/Constant  arith_type=Unsigned  const=0  n_bits=18  bin_pt=17  explicit_period=off  period=1  equ=P=C  opselect=C  inp2=PCIN>>17  opr=+  inp1=P  carry=CIN  dbl_ovrd=off  block_type=constant
      settings: block_version=11.4
  sync_out : Outport
  dout : Outport  Port=2
  wires:
  sync/1 -> sync_delay/1
  sync_delay/1 -> sync_out/1

== system xblock_half_band_Model/Subsystem/parallel_fir/f1/fir_col1 ==
  real1 : Inport
  imag1 : Inport  Port=2
  fir_tap1 : Subsystem
  real_out1 : Outport
  imag_out1 : Outport  Port=2
  real_sum : Outport  Port=3
  imag_sum : Outport  Port=4
  wires:
  fir_tap1/4(imag) -> imag_sum/1  "xlsub5_fir_tap1_image"
  fir_tap1/1(a_out) -> real_out1/1
  real1/1 -> fir_tap1/1(a)
  imag1/1 -> fir_tap1/2(b)
  fir_tap1/2(b_out) -> imag_out1/1
  fir_tap1/3(real) -> real_sum/1  "xlsub5_fir_tap1_real"

== system xblock_half_band_Model/Subsystem/parallel_fir/f1/fir_col2 ==
  real1 : Inport
  imag1 : Inport  Port=2
  fir_tap1 : Subsystem
  real_out1 : Outport
  imag_out1 : Outport  Port=2
  real_sum : Outport  Port=3
  imag_sum : Outport  Port=4
  wires:
  fir_tap1/4(imag) -> imag_sum/1  "xlsub5_fir_tap1_image"
  fir_tap1/1(a_out) -> real_out1/1
  real1/1 -> fir_tap1/1(a)
  imag1/1 -> fir_tap1/2(b)
  fir_tap1/2(b_out) -> imag_out1/1
  fir_tap1/3(real) -> real_sum/1  "xlsub5_fir_tap1_real"

== system xblock_half_band_Model/Subsystem/parallel_fir/f1/fir_col3 ==
  real1 : Inport
  imag1 : Inport  Port=2
  fir_tap1 : Subsystem
  real_out1 : Outport
  imag_out1 : Outport  Port=2
  real_sum : Outport  Port=3
  imag_sum : Outport  Port=4
  wires:
  fir_tap1/4(imag) -> imag_sum/1  "xlsub5_fir_tap1_image"
  fir_tap1/1(a_out) -> real_out1/1
  real1/1 -> fir_tap1/1(a)
  imag1/1 -> fir_tap1/2(b)
  fir_tap1/2(b_out) -> imag_out1/1
  fir_tap1/3(real) -> real_sum/1  "xlsub5_fir_tap1_real"

== system xblock_half_band_Model/Subsystem/parallel_fir/f1/fir_col4 ==
  real1 : Inport
  imag1 : Inport  Port=2
  fir_tap1 : Subsystem
  real_out1 : Outport
  imag_out1 : Outport  Port=2
  real_sum : Outport  Port=3
  imag_sum : Outport  Port=4
  wires:
  fir_tap1/4(imag) -> imag_sum/1  "xlsub5_fir_tap1_image"
  fir_tap1/1(a_out) -> real_out1/1
  real1/1 -> fir_tap1/1(a)
  imag1/1 -> fir_tap1/2(b)
  fir_tap1/2(b_out) -> imag_out1/1
  fir_tap1/3(real) -> real_sum/1  "xlsub5_fir_tap1_real"

== system xblock_half_band_Model/Subsystem/parallel_fir/f1/fir_col5 ==
  real1 : Inport
  imag1 : Inport  Port=2
  fir_tap1 : Subsystem
  real_out1 : Outport
  imag_out1 : Outport  Port=2
  real_sum : Outport  Port=3
  imag_sum : Outport  Port=4
  wires:
  fir_tap1/4(imag) -> imag_sum/1  "xlsub5_fir_tap1_image"
  fir_tap1/1(a_out) -> real_out1/1
  real1/1 -> fir_tap1/1(a)
  imag1/1 -> fir_tap1/2(b)
  fir_tap1/2(b_out) -> imag_out1/1
  fir_tap1/3(real) -> real_sum/1  "xlsub5_fir_tap1_real"

== system xblock_half_band_Model/Subsystem/parallel_fir/f1/fir_col6 ==
  real1 : Inport
  imag1 : Inport  Port=2
  fir_tap1 : Subsystem
  real_out1 : Outport
  imag_out1 : Outport  Port=2
  real_sum : Outport  Port=3
  imag_sum : Outport  Port=4
  wires:
  fir_tap1/4(imag) -> imag_sum/1  "xlsub5_fir_tap1_image"
  fir_tap1/1(a_out) -> real_out1/1
  real1/1 -> fir_tap1/1(a)
  imag1/1 -> fir_tap1/2(b)
  fir_tap1/2(b_out) -> imag_out1/1
  fir_tap1/3(real) -> real_sum/1  "xlsub5_fir_tap1_real"

== system xblock_half_band_Model/Subsystem/parallel_fir/f1/fir_col7 ==
  real1 : Inport
  imag1 : Inport  Port=2
  fir_tap1 : Subsystem
  real_out1 : Outport
  imag_out1 : Outport  Port=2
  real_sum : Outport  Port=3
  imag_sum : Outport  Port=4
  wires:
  fir_tap1/4(imag) -> imag_sum/1  "xlsub5_fir_tap1_image"
  fir_tap1/1(a_out) -> real_out1/1
  real1/1 -> fir_tap1/1(a)
  imag1/1 -> fir_tap1/2(b)
  fir_tap1/2(b_out) -> imag_out1/1
  fir_tap1/3(real) -> real_sum/1  "xlsub5_fir_tap1_real"

== system xblock_half_band_Model/Subsystem/parallel_fir/f1/fir_col8 ==
  real1 : Inport
  imag1 : Inport  Port=2
  fir_tap1 : Subsystem
  real_out1 : Outport
  imag_out1 : Outport  Port=2
  real_sum : Outport  Port=3
  imag_sum : Outport  Port=4
  wires:
  fir_tap1/4(imag) -> imag_sum/1  "xlsub5_fir_tap1_image"
  fir_tap1/1(a_out) -> real_out1/1
  real1/1 -> fir_tap1/1(a)
  imag1/1 -> fir_tap1/2(b)
  fir_tap1/2(b_out) -> imag_out1/1
  fir_tap1/3(real) -> real_sum/1  "xlsub5_fir_tap1_real"
